simulink model "zad3_model"  (R2023a)
settings: Solver=VariableStepAuto  StartTime=0.0  StopTime=8  RelTol=1e-3
values from neighbouring files (symbols this model uses):
  a1 = Gz.Numerator{1}(2)    [zad1.m]
  a2 = Gz.Numerator{1}(3)    [zad1.m]
  a3 = Gz.Numerator{1}(4)    [zad1.m]
  b0 = Gz.Denominator{1}(1)    [zad1.m]
  b1 = Gz.Denominator{1}(2)    [zad1.m]
  b2 = Gz.Denominator{1}(3)    [zad1.m]
  b3 = Gz.Denominator{1}(4)    [zad1.m]
  T = 0.5    [zad1.m]
settings Model: Creator=denys  LastModifiedBy=denys

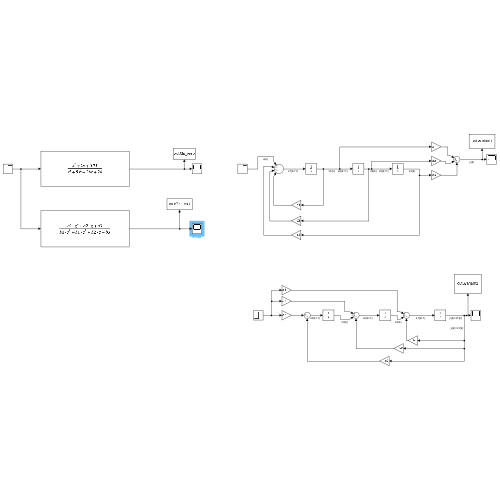
[thumbnail: Simulink's stored preview of the top-level diagram]
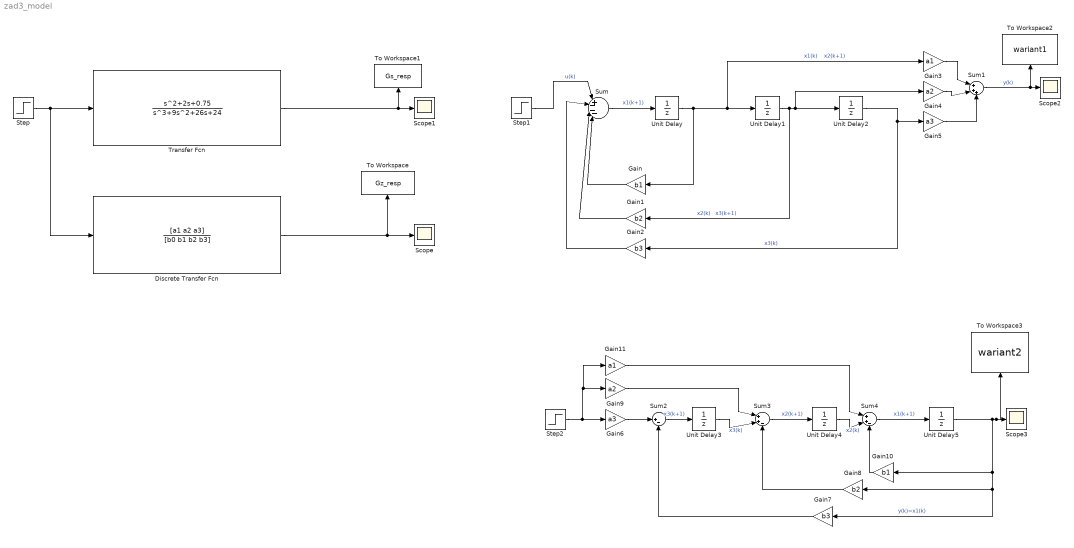
== system zad3_model ==
  Discrete Transfer Fcn : DiscreteTransferFcn  Numerator=[a1 a2 a3]  Denominator=[b0 b1 b2 b3]
  Gain : Gain  Gain=b1
  Gain1 : Gain  Gain=b2
  Gain10 : Gain  Gain=b1
  Gain11 : Gain  Gain=a1
  Gain2 : Gain  Gain=b3
  Gain3 : Gain  Gain=a1
  Gain4 : Gain  Gain=a2
  Gain5 : Gain  Gain=a3
  Gain6 : Gain  Gain=a3
  Gain7 : Gain  Gain=b3
  Gain8 : Gain  Gain=b2
  Gain9 : Gain  Gain=a2
  Scope{,1..3} (4 alike) : Scope
  Step : Step  SampleTime=T
  Step1 : Step  SampleTime=T
  Step2 : Step  SampleTime=T
  Sum : Sum  Inputs=|+---|
  Sum1 : Sum  Inputs=|+++
  Sum2 : Sum  Inputs=|+-
  Sum3 : Sum  Inputs=|++-
  Sum4 : Sum  Inputs=|++-
  To Workspace : ToWorkspace  VariableName=Gz_resp  SaveFormat=Timeseries  SampleTime=T
  To Workspace1 : ToWorkspace  VariableName=Gs_resp  SaveFormat=Timeseries  SampleTime=-1
  To Workspace2 : ToWorkspace  VariableName=wariant1  SaveFormat=Timeseries  SampleTime=T
  To Workspace3 : ToWorkspace  VariableName=wariant2  SaveFormat=Timeseries  SampleTime=T
  Transfer Fcn : TransferFcn  Numerator=[1 2 0.75]  Denominator=[1 9 26 24]
  Unit Delay{,1..5} (6 alike) : UnitDelay  SampleTime=-1  HasFrameUpgradeWarning=on
  wires:
  Transfer Fcn/1 -> To Workspace1/1, Scope1/1
  Discrete Transfer Fcn/1 -> Scope/1, To Workspace/1
  Step/1 -> Discrete Transfer Fcn/1, Transfer Fcn/1
  Gain5/1 -> Sum1/3
  Gain2/1 -> Sum/2
  Sum1/1 -> Scope2/1, To Workspace2/1  "y(k)"
  Unit Delay/1 -> Gain3/1, Unit Delay1/1, Gain/1  "x1(k)    x2(k+1)"
  Gain1/1 -> Sum/3
  Gain/1 -> Sum/4
  Step1/1 -> Sum/1  "u(k)"
  Sum/1 -> Unit Delay/1  "x1(k+1)"
  Gain4/1 -> Sum1/2
  Unit Delay1/1 -> Unit Delay2/1, Gain4/1, Gain1/1  "x2(k)   x3(k+1)"
  Unit Delay2/1 -> Gain2/1, Gain5/1  "x3(k)"
  Gain3/1 -> Sum1/1
  Gain10/1 -> Sum4/3
  Gain6/1 -> Sum2/1
  Sum4/1 -> Unit Delay5/1  "x1(k+1)"
  Sum2/1 -> Unit Delay3/1  "x3(k+1)"
  Unit Delay4/1 -> Sum4/2  "x2(k)"
  Gain7/1 -> Sum2/2
  Sum3/1 -> Unit Delay4/1  "x2(k+1)"
  Gain11/1 -> Sum4/1
  Step2/1 -> Gain11/1, Gain9/1, Gain6/1
  Gain9/1 -> Sum3/1
  Unit Delay3/1 -> Sum3/2  "x3(k)"
  Unit Delay5/1 -> To Workspace3/1, Scope3/1, Gain10/1, Gain7/1, Gain8/1  "y(k)=x1(k)"
  Gain8/1 -> Sum3/3
